simulink model "sim_all"  (R2020a)
settings: Solver=VariableStepAuto  StartTime=0.0  StopTime=2000  RelTol=1e-3
values from neighbouring files (symbols this model uses):
  a1 = rho * D^4 * alpha1    (= 0.000388302366464)    [data_current.m]
  a2 = -rho * D^3 * alpha2 * (1 - omega)    (= 0.0037030698432)    [data_current.m]
  alpha1 = 0.0113    [data_current.m]
  alpha2 = -0.0091    [data_current.m]
  cornerA = [43.781381 ... (first row only)    [missionC.m]
  cornerB = [43.780975 ... (first row only)    [missionC.m]
  cornerC = [43.780189 ... (first row only)    [missionC.m]
  cornerD = [43.780602 ... (first row only)    [missionC.m]
  ctrl_clockwise = false    [controller.m]
  ctrl_int_bound_or = 0.1    [controller.m]
  ctrl_int_bound_pos = 1    [controller.m]
  ctrl_k_or = 1    [controller.m]
  ctrl_k_pos = 1/3    (= 0.333333333333)    [controller.m]
  ctrl_Ki_vel = 100    [controller.m]
  ctrl_Kp_v_pos = 200    [controller.m]
  ctrl_Kp_vel = 200    [controller.m]
  ctrl_TAM = [  1     1           0           0               0       0;               0     0           1           1               0       0;               0     0           0           0               1       1;               0     0  -(ctrl_r+ctrl_dc)  ctrl_r+ctrl_dc    0       0;               0     0           0           0            -ctrl_r    ctrl_r;           -ctrl_r ctrl_r        0           0       ...(+19 chars)    [controller.m]
  ctrl_Ts = 0.1    [controller.m]
  ctrl_va_uncontrolled = 0.15    [controller.m]
  ctrl_vel_uncontrolled = 0.5    [controller.m]
  D = 0.076    [data_current.m]
  dead_zone_limit = 31.5    [data_current.m]
  depth = 5    [missionC.m]
  distanceFromWall = 8    [missionC.m]
  initInspectedSide = 2    [missionC.m]
  initPoint = [ 43.780796 ... (first row only)    [missionC.m]
  mod_A = pi*mod_R*mod_R    [model.m]
  mod_Cd_F = 0.45    [model.m]
  mod_Cd_M = 0.4    [model.m]
  mod_eta_init = [mod_xNorth; mod_yEast; -mod_zDown; 0; 0; 0]    [model.m]
  mod_g = 9.81    [model.m]
  mod_h0 = 0    [model.m]
  mod_Ixx = mod_Io(1,1)    [model.m]
  mod_Iyy = mod_Io(2,2)    [model.m]
  mod_Izz = mod_Io(3,3)    [model.m]
  mod_Kp_dot = 0    [model.m]
  mod_lat0 = 43.780189    [model.m]
  mod_lon0 = 11.282698    [model.m]
  mod_m = 100    [model.m]
  mod_Mq_dot = mod_Kp_dot    (= 0)    [model.m]
  mod_ni_init = [0; 0; 0; 0; 0; 0]    [model.m]
  mod_Nr_dot = mod_Kp_dot    (= 0)    [model.m]
  mod_p1 = [0; mod_R; 0]    [model.m]
  mod_p2 = [0; -mod_R; 0]    [model.m]
  mod_p3 = [0; 0; (mod_R + mod_z_cm)]    [model.m]
  mod_p4 = [0; 0; -(mod_R + mod_z_cm)]    [model.m]
  mod_p5 = [mod_R; 0; 0]    [model.m]
  mod_p6 = [-mod_R; 0; 0]    [model.m]
  mod_R = ((3*mod_Vol)/(4*pi))^(1/3)    [model.m]
  mod_Rm = (4*mod_R)/(3*pi)    [model.m]
  mod_t1 = [1; 0; 0]    [model.m]
  mod_t2 = [1; 0; 0]    [model.m]
  mod_t3 = [0; 1; 0]    [model.m]
  mod_t4 = [0; 1; 0]    [model.m]
  mod_t5 = [0; 0; 1]    [model.m]
  mod_t6 = [0; 0; 1]    [model.m]
  mod_W = mod_m*mod_g    (= 981)    [model.m]
  mod_Xu_dot = (2/3)*mod_rho_AUV*pi*(mod_R^3)    [model.m]
  mod_Yv_dot = mod_Xu_dot    [model.m]
  mod_z_cm = mod_r_cm(3)    [model.m]
  mod_Zw_dot = mod_Xu_dot    [model.m]
  n_max = 340    [data_current.m]
  nav_DT = 0.1    [navigation.m]
  nav_filter = -1    [data_analysis_simulation_total.m]    (also in navigation.m)
  nav_giro = 2    [navigation.m]
  nav_h0 = 0    [navigation.m]
  nav_lat0 = cornerC(1)    [navigation.m]
  nav_lon0 = cornerC(2)    [navigation.m]
  nav_plane_AB = coefficient_plane(nav_A,nav_B)    [navigation.m]
  nav_plane_BC = coefficient_plane(nav_B,nav_C)    [navigation.m]
  nav_plane_CD = coefficient_plane(nav_C,nav_D)    [navigation.m]
  nav_plane_DA = coefficient_plane(nav_D,nav_A)    [navigation.m]
  nav_resampling = 10000    [navigation.m]
  omega = 0.1    [data_current.m]
  relativeDirection = 30    [missionC.m]
  res_enable_n_eff = 1    [navigation.m]
  rho = 1030    [data_current.m]
  sens_distCM = 0.267    [sensors.m]
  sens_Sample_time_AHRS = 0.1    [sensors.m]
  sens_Sample_time_depth = 0.1    [sensors.m]
  sens_Sample_time_dvl = 0.2    [sensors.m]
  sens_Sample_time_GPS = 1    [sensors.m]
  sens_Sample_time_GYRO = 0.1    [sensors.m]
  sens_Sample_time_sonar = 0.5    [sensors.m]
  sens_threshold = 0.485    [sensors.m]
  sens_Variance_AHRS_pitch = (0.0087)^2    (= 7.569e-05)    [sensors.m]
  sens_Variance_AHRS_roll = (0.0087)^2    (= 7.569e-05)    [sensors.m]
  sens_Variance_AHRS_yaw = (0.0017)^2    (= 2.89e-06)    [sensors.m]
  sens_Variance_depth1 = (0.2)^2    (= 0.04)    [sensors.m]
  sens_Variance_depth2 = (0.4)^2    (= 0.16)    [sensors.m]
  sens_Variance_DVL = (speed*0.03)^2    [sensors.m]
  sens_Variance_GPS = 3    [sensors.m]
  sens_Variance_GYRO = 2.5133e-06    [sensors.m]
  sens_Variance_sonar = 0.05    [sensors.m]
  soglia_or = [0.1, 0.1, 0.1]    [mission.m]
  soglia_orp = 0.1    [mission.m]
  soglia_parete = 0.5    [mission.m]
  soglia_parete_frenata = 0.5    [mission.m]
  soglia_pos = [0.00001, 0.00001, 0.5]    [mission.m]
  soglia_SOS_collisione = 2    [mission.m]
  soglia_SOS_or = [0.25, 0.25, 0.25]    [mission.m]
  soglia_SOS_orp = 0.25    [mission.m]
  soglia_SOS_parete = 1    [mission.m]
  soglia_SOS_pos = [0.00005, 0.00005, 1]    [mission.m]
  soglia_SOS_pos_ris = 2    [mission.m]
  soglia_SOS_vel = 0.2    [mission.m]
  SOS = 0    [mission.m]
  speed = 0.4    [missionC.m]
  stato = 100    [mission.m]
  timer = 40*2    (= 80)    [mission.m]
  Ts_supervisor = 0.1    [mission.m]
undefined symbols (not defined in the file or in its folder): DiscIntNeverNeededParam, nav_A, nav_B, nav_C, nav_D
libraries: simulink x8, cstblocks x6, simulink_extras x1
(part 7 of 8)

== matlab function sim_all/Controller_mk4_v3/C_or/C_or_Z ==
  data: err_int output; ang input; vel output; k input; ctrl_va_uncontrolled parameter; ctrl_int_bound_or parameter
%% Azione proporzionale
function [err_int, vel] = fcn(ang, k, ctrl_va_uncontrolled, ctrl_int_bound_or)
    v = 0;
    err_int = 0;
    va_des = ctrl_va_uncontrolled;  % velocità impostata prima della fase di frenata
    brake_dist = (1/k)*va_des;      % distanza in cui dobbiamo iniziare a frenare
    if ang >= brake_dist            % al di fuori dello spazio di frenata
        v = va_des;
    end
    if ang <= -brake_dist           % al di fuori dello spazio di frenata in negativo
        v = -va_des;
    end
    if  abs(ang) < brake_dist       % proporzionale se entro la distanza di frenata
        v = k*ang;
    end
    vel = v;
    if abs(ang) < ctrl_int_bound_or    % per il regime può essere utile una azione integrale
        err_int = ang;                 % err_int va ad un integratore
    end
end

== matlab function sim_all/Controller_mk4_v3/C_pos/C_pos_X ==
  data: err_int output; pos input; vel output; k input; ctrl_vel_uncontrolled parameter; ctrl_int_bound_pos parameter
%% Azione proporzionale
function [err_int, vel] = fcn(pos, k, ctrl_vel_uncontrolled, ctrl_int_bound_pos)
    v = 0;
    err_int = 0;
    vel_des = ctrl_vel_uncontrolled;    % velocità impostata se 'lontani'
    brake_dist = 1/k*vel_des;           % distanza di frenata
    if pos >= brake_dist                % se ho spazio per frenare mantengo la velocità
        v = vel_des;
    end
    if pos <= -brake_dist               % lontani in direzione negativa
        v = -vel_des;
    end
    if  abs(pos) < brake_dist           % se è vicino il proporzionale gestisce la frenata
        v = k*pos;
    end
    vel = v;
    if abs(pos) < ctrl_int_bound_pos    % per il regime può essere utile una azione integrale
        err_int = pos;                  % err_int va ad un integratore
    end

== matlab function sim_all/Controller_mk4_v3/C_pos/C_pos_Z ==
  data: err_int output; pos input; vel output; k input; ctrl_vel_uncontrolled parameter; ctrl_int_bound_pos parameter
%% Azione proporzionale
function [err_int, vel] = fcn(pos, k, ctrl_vel_uncontrolled, ctrl_int_bound_pos)
    v = 0;
    err_int = 0;
    vel_des = ctrl_vel_uncontrolled;    % velocità impostata se 'lontani'
    brake_dist = 1/k*vel_des;           % distanza di frenata
    if pos >= brake_dist                % se ho spazio per frenare mantengo la velocità
        v = vel_des;
    end
    if pos <= -brake_dist               % lontani in direzione negativa
        v = -vel_des;
    end
    if  abs(pos) < brake_dist           % se è vicino il proporzionale gestisce la frenata
        v = k*pos;
    end
    vel = v;
    if abs(pos) < ctrl_int_bound_pos    % per il regime può essere utile una azione integrale
        err_int = pos;                  % err_int va ad un integratore
    end

== matlab function sim_all/PF/Particle Filter/AHRS__check/MATLAB Function4 ==
  data: flag_AHRS output; AHRS_new input; AHRS_now output; AHRS_old input
function [flag_AHRS, AHRS_now] = fcn(AHRS_new, AHRS_old)

    if isnan(AHRS_new(1,1)) || isnan(AHRS_new(2,1)) || isnan(AHRS_new(3,1))
        AHRS_now = AHRS_old;
        flag_AHRS = 1;
        disp('Misura AHRS non valida')
    else
        AHRS_now = AHRS_new;
        flag_AHRS = 0;
    end  
end

== matlab function sim_all/PF/Particle Filter/CORREZIONE/MATLAB Function ==
  data: x_k_1 input; x output; P_k_1 input; s input size=3 1000; w input size=1 1000; flag input; P output; s output; w output; nav_flag_init input
function [x, P, s, w] = correction(x_k_1, P_k_1, s, w, flag,nav_flag_init)

%% -------------------------------------------
    n=1000; 
%% -------------------------------------------

%in base al flag so se i pesi sono stati aggionati o meno nella correzione
%e quindi decido se ricalcolare le x stimate e la P oppure no
       
    x=zeros(3,1); 
    P=zeros(3,3);

    if nav_flag_init ~= 0       %se il filtro è inizializzato
        if flag == 1            %se la correzione è avvenuta ricalcolo x e P
            for i=1:3
                x(i) = sum(w(1,:)*s(i,:)');
            end
            for i=1:n   
              P = P + w(:,i)*((s(:,i)-x)*(s(:,i)-x)');  
            end
        else                    % se la correzione è avvenuta
            x=x_k_1;
            P=P_k_1;
        end
    end
end

== matlab function sim_all/PF/Particle Filter/Creazione vettore delle misure ==
  data: flag_vect output; GPS input; mis_vect output; depth input; s_pr input; s_dx input; s_sx input; mis_vect_prec input; J input; pos input; nav_plane_AB parameter; nav_plane_BC parameter; nav_plane_CD parameter; nav_plane_DA parameter; nav_A parameter; nav_B parameter; nav_C parameter; nav_D parameter; distanceFromWall parameter
%%
% Questa funzione impila le informazioni derivanti dai vari sensori in un
% unico vettore mis_vect 7x1.                                 
% Ci sarà un corrispondente vettore flag_vect 7x1 di flag che sarà pari a:

% flag(i) = 0  se la misura è uguale a quella arrivata nell'istante
% predecente, in tal caso la correzione non verrà effettuata
% flag(i) = 1 se la misura è stata aggiornata rispetto a quella precendente
 
% NB il controllo sulla validità dei dati del GPS è valutata nel blocco
% sucessivo

function [flag_vect,mis_vect] = misure_vector(GPS,depth,s_pr,s_dx,s_sx, mis_vect_prec,...
          J,pos, nav_plane_AB, nav_plane_BC, nav_plane_CD, nav_plane_DA, nav_A, nav_B, nav_C, nav_D, distanceFromWall)
    
    mis_vect = zeros(7,1);
    flag_vect = zeros(7,1);
	mis_vect = [GPS(1) GPS(2) GPS(3) depth s_pr s_dx s_sx]';
    
    for i=[1:7]
        if mis_vect(i) ~= mis_vect_prec(i)
            flag_vect(i) = 1;
        end
    end
    
    %valutiamo se la misura del profondimetro è valida
    if isnan(depth)  
        flag_vect(4) = 0;
    end
     
    %se i dati dei sonar qui sono utilizzabili, dobbiamo assicurarci che il 
    %loro raggio non punti verso uno spigolo, in quel caso potrebbe
    %causare una correzione errata
    
    if flag_vect(5) == 1               %se i dati del sonar di prua sono nuovi
            versore_son_NED = J*[1 0 0]';          %versore terna NED sonar prua
            flag_vect(5) = inter(pos, versore_son_NED ,nav_plane_AB,nav_plane_BC,nav_plane_CD,nav_plane_DA, nav_A, nav_B, nav_C, nav_D);       
    end

    if flag_vect(6) == 1               %se i dati del sonar destro sono nuovi
            versore_son_NED = J*[0 1 0]';          %versore terna NED sonar dx

            flag_vect(6) = inter(pos, versore_son_NED ,nav_plane_AB,nav_plane_BC,nav_plane_CD,nav_plane_DA, nav_A, nav_B, nav_C, nav_D);       
    end
    if flag_vect(7) == 1               %se i dati del sonar sinistro sono nuovi
            versore_son_NED = J*[0 -1 0]';          %versore terna NED sonar sx
            flag_vect(7) = inter(pos, versore_son_NED ,nav_plane_AB,nav_plane_BC,nav_plane_CD,nav_plane_DA, nav_A, nav_B, nav_C, nav_D);
    end 
    %la terza componente di flag_vect non sarà utilizzata. per assicurarci
    %che i dati del GPS siano validi ci rifaremo sempre su mis_vect
    
    
    
    %se il valore del sonar è NaN, non dobbiamo considerare valide le
    %misure, e se il robot troppo lontane dalle pareti
    soglia_distanza=distanceFromWall*3;
    soglia_variazione=0.8;
    if isnan(s_pr) || mis_vect(5) > soglia_distanza || abs(mis_vect(5)- mis_vect_prec(5)) > soglia_variazione
        flag_vect(5) = 0;
    end
    if isnan(s_dx) || mis_vect(6) > soglia_distanza || abs(mis_vect(6)- mis_vect_prec(6)) > soglia_variazione
        flag_vect(6) = 0;
    end
    if isnan(s_sx) || mis_vect(7) > soglia_distanza || abs(mis_vect(7)- mis_vect_prec(7)) > soglia_variazione
        flag_vect(7) = 0;
    end
end




function [flag] = inter(pos, versore_son_NED,nav_plane_AB,nav_plane_BC,nav_plane_CD,nav_plane_DA, nav_A, nav_B, nav_C, nav_D)
    
    %calcolo della distanza dalla posizione ai piani delle pareti seguendo
    %la direzione data dal versore del sonar

    t_AB = -(pos(1)+nav_plane_AB(2)*pos(2)+nav_plane_AB(4))/(nav_plane_AB(2)*versore_son_NED(2)+versore_son_NED(1));
    t_BC = -(pos(1)+nav_plane_BC(2)*pos(2)+nav_plane_BC(4))/(nav_plane_BC(2)*versore_son_NED(2)+versore_son_NED(1));
    t_CD = -(pos(1)+nav_plane_CD(2)*pos(2)+nav_plane_CD(4))/(nav_plane_CD(2)*versore_son_NED(2)+versore_son_NED(1));
    t_DA = -(pos(1)+nav_plane_DA(2)*pos(2)+nav_plane_DA(4))/(nav_plane_DA(2)*versore_son_NED(2)+versore_son_NED(1));
    
    if t_AB < 0
        t_AB = inf;
    end
    if t_BC < 0
        t_BC = inf;
    end
    if t_CD < 0
        t_CD = inf;
    end
    if t_DA < 0
        t_DA = inf;
    end
           
    [dist, index] = min([t_AB t_BC t_CD t_DA]);
    dist = dist - 0.267;       %va tolto il raggio del robot rispetto al centro di massa
    
    int=zeros(1,3);
    %calcolo l'intersezione
    int(1) = pos(1) + versore_son_NED(1)*dist;
    int(2) = pos(2) + versore_son_NED(2)*dist;
    int(3) = 0;
    
    
    
    soglia_spigolo = 5;          %distanza massima dallo spigolo entro la quale 
                       %la misura del sonar non è buona
    flag=1;
    switch index
        case 1      
            if norm(int-nav_A) < soglia_spigolo || norm(int-nav_B) < soglia_spigolo
                flag=0;
            end
        case 2
            if norm(int-nav_B) < soglia_spigolo || norm(int-nav_C) < soglia_spigolo
                flag=0;
            end
        case 3
            if norm(int-nav_C) < soglia_spigolo || norm(int-nav_D) < soglia_spigolo
                flag=0;
            end
        case 4
            if norm(int-nav_D) < soglia_spigolo || norm(int-nav_A) < soglia_spigolo
                flag=0;
            end
        otherwise
            disp('errore nella intersezione del piano')
    end
end

== matlab function sim_all/Mission_supervisor_v3/Mission_Supervisor/MATLAB Function1 ==
  data: punto_iniz_patt output size=3; initInspectedSide parameter; distanceFromWall parameter; initPoint parameter; Or_in output; dps_fin output; cornerA parameter; cornerB parameter; cornerC parameter; cornerD parameter; relativeDirection parameter; alfa output
function [punto_iniz_patt, Or_in, dps_fin, alfa] = ambiente(initInspectedSide,distanceFromWall,initPoint,cornerA, cornerB, cornerC, cornerD, relativeDirection)
 
    %% Unità di misura 
    
    % punto_iniz_patt, initPoint, cornerA, cornerB, cornerC, cornerD        [deg, deg, m]
    % Or_in                                                                 [rad, rad, rad]
    % dps_fin,distanceFromWall                                              [m]
    % alfa                                                                  [rad]
    % relativeDirection                                                     [deg]

    %% Inizializzazione variabili
    
    % Valori dati da file relativi agli angoli del bacino
    iP = initPoint;
    A = cornerA;
    B = cornerB;
    C = cornerC;
    D = cornerD;

    coder.extrinsic('evalin', 'wgs84Ellipsoid', 'geodetic2ned');
    coder.extrinsic('evalin', 'wgs84Ellipsoid', 'ned2geodetic');

    % Inizializzazione di alcune variabili
    xA = 0; yA = 0; zA = 0; xB = 0; yB = 0; zB = 0; xC = 0; yC = 0; zC = 0; 
    xD = 0; yD = 0; zD = 0; xiP = 0; yiP = 0; ziP = 0;
    xpipAB = 0; ypipAB = 0; zpipAB = 0; xpipBC = 0; ypipBC = 0; zpipBC = 0; 
    xpipCD = 0; ypipCD = 0; zpipCD = 0; xpipDA = 0; ypipDA = 0; zpipDA = 0;
    depth_in = initPoint(3);
    Or_in = [0; 0; 0];
    
    % Conversione da Geodetic a NED delle posizioni degli angoli e del punto iniziale
    wgs84 = wgs84Ellipsoid; % Per il corretto funzionamento e' necessario installare un 
                            % pacchetto aggiuntivo in Matlab qualora non fosse presente
    [xA, yA, zA] = geodetic2ned(A(1), A(2), 0, C(1), C(2), 0, wgs84);
    [xB, yB, zB] = geodetic2ned(B(1), B(2), 0, C(1), C(2), 0, wgs84);
    [xC, yC, zC] = geodetic2ned(C(1), C(2), 0, C(1), C(2), 0, wgs84);
    [xD, yD, zD] = geodetic2ned(D(1), D(2), 0, C(1), C(2), 0, wgs84);
    [xiP, yiP, ziP] = geodetic2ned(iP(1), iP(2), 0, C(1), C(2), 0, wgs84);
    inizio = [xiP; yiP; depth_in];

    % Punti centrali delle pareti
    pcAB = [(xB + xA)/2; (yB + yA)/2; depth_in];
    pcBC = [(xB + xC)/2; (yB + yC)/2; depth_in];   
    pcCD = [(xC + xD)/2;(yC + yD)/2; depth_in];
    pcDA = [(xD + xA)/2; (yD + yA)/2; depth_in];

    % Lunghezze delle pareti
    AB = sqrt((xA - xB)^2 + (yA - yB)^2); 
    BC = sqrt((xB - xC)^2 + (yB - yC)^2); 
    CD = sqrt((xC - xD)^2 + (yC - yD)^2); 
    DA = sqrt((xD - xA)^2 + (yD - yA)^2); 
    
    dW = distanceFromWall;

    %% Calcolo punto di inizio pattugliamento a meta' parete

    % Calcolo degli angoli relativi tra le pareti 
    thetaBC = acos(yB/BC);          
    thetaCD = acos(yD/CD);
    gammaAB = acos((yB - yA)/AB);
    thetaAB = pi - gammaAB;
    gammaDA = acos((yA - yD)/DA);

    % Punti di inizio pattugliamento a seconda di quale parete è scelta come
    % parete iniziale
    
    dbpc = sqrt((pcAB(1) - xB)^2 + (pcAB(2) - yB)^2);
    hpb = sqrt(dbpc^2 + dW^2);
    alfa1 = - acos(dbpc/hpb);
    gammaab = pi - (gammaAB + alfa1);
    pcab1 = [hpb * sin(gammaab), hpb * cos(gammaab)];
    pipAB = [xB + pcab1(1); yB + pcab1(2); depth_in];

    dcpc = sqrt(pcBC(1)^2 + pcBC(2)^2);
    hpc = sqrt(dcpc^2 + dW^2);
    alfabc = acos(dcpc/hpc);
    gammaBC = thetaBC + alfabc;
    pipBC = [hpc * sin(gammaBC); hpc * cos(gammaBC); depth_in];

    dcdpc = sqrt(pcCD(1)^2 + pcCD(2)^2);
    hpcd = sqrt(dcdpc^2 + dW^2);
    alfacd = acos(dcdpc/hpcd);
    gammaCD = thetaCD - alfacd;
    pipCD = [hpcd * sin(gammaCD); hpcd * cos(gammaCD); depth_in];

    dapc = sqrt((pcDA(1) - xA)^2 + (pcDA(2) - yA)^2);
    hpda = sqrt(dapc^2 + dW^2);
    alfada = acos(dapc/hpda);
    gammada = pi + (gammaDA + alfada);
    pcda1 = [hpda * sin(gammada), hpda * cos(gammada)];
    pipDA = [xA + pcda1(1); yA + pcda1(2); depth_in];
    
    % Si convertono i punti "pip" da NED a Geodetic 
    [xpipAB, ypipAB, zpipAB] = ned2geodetic(pipAB(1), pipAB(2), pipAB(3), C(1), C(2), 0, wgs84);
    [xpipBC, ypipBC, zpipBC] = ned2geodetic(pipBC(1), pipBC(2), pipBC(3), C(1), C(2), 0, wgs84);
    [xpipCD, ypipCD, zpipCD] = ned2geodetic(pipCD(1), pipCD(2), pipCD(3), C(1), C(2), 0, wgs84);
    [xpipDA, ypipDA, zpipDA] = ned2geodetic(pipDA(1), pipDA(2), pipDA(3), C(1), C(2), 0, wgs84);

    pipAB_geodetic = [xpipAB; ypipAB; depth_in];
    pipBC_geodetic = [xpipBC; ypipBC; depth_in];
    pipCD_geodetic = [xpipCD; ypipCD; depth_in];
    pipDA_geodetic = [xpipDA; ypipDA; depth_in];

    %% Calcolo angolo di orientazione iniziale in direzione del punto di inizio  pattugliamento (rispetto al nord)

    % Versore orinetato verso il nord n = [1, 0, 0];
    
    % Vettori che vanno dal punto di partenza al punto di inizio pattugliamento
    
    iAB = pipAB - inizio;
    iBC = pipBC - inizio;
    iCD = pipCD - inizio;
    iDA = pipDA - inizio;

    % Angoli tra direzione Nord e il vettore che porta verso il punto di inizio pattugliamento. 
    % Sono gli angoli di orientazione iniziale desiderata. 
    theta1 = atan2d(iAB(2),iAB(1));
    theta2 = atan2d(iBC(2),iBC(1));
    theta3 = atan2d(iCD(2),iCD(1));
    theta4 = atan2d(iDA(2),iDA(1));
    
    % Si raccoglie in un vettore
    theta = [deg2rad(theta1), deg2rad(theta2), deg2rad(theta3), deg2rad(theta4)];

    %% Si calcolano gli angoli interni dei vertici
    
    alfaC = thetaCD - thetaBC;
    alfaB = pi - (thetaAB-thetaBC);
    alfaA = thetaAB - gammaDA;
    alfaD = 2*pi - alfaA - alfaB - alfaC;
    alfa = [alfaA; alfaB; alfaC; alfaD];    %Utilizzati poi in fase di manovra

    %% Calcolo distanza dalla parete successiva a partire da meta'  parete

    % Sono le distanze da metà parete alla parete successiva
    dABpc = sqrt((pcAB(1) - xB)^2 + (pcAB(2) - yB)^2);
    dBCpc = sqrt(pcBC(1)^2 + pcBC(2)^2);
    dCDpc = sqrt(pcCD(1)^2 + pcCD(2)^2);
    dDApc = sqrt((pcDA(1) - xA)^2 + (pcDA(2) - yA)^2);


    %% Scelta delle condizioni

    % In base al valore di parete iniziale si assegnano i giusti valori per i 
    % riferimenti da utilizzare nei vari stati
    
    if initInspectedSide == 1

        punto_iniz_patt = pipAB_geodetic;
        Or_in = [0; 0; theta(1)];
        dps_fin = dABpc;

    elseif initInspectedSide == 2

        punto_iniz_patt = pipBC_geodetic;
        Or_in = [0; 0; theta(2)];
        dps_fin = dBCpc;

    elseif initInspectedSide == 3

        punto_iniz_patt = pipCD_geodetic;
        Or_in = [0; 0; theta(3)];
        dps_fin = dCDpc;

    else

        punto_iniz_patt = pipDA_geodetic;
        Or_in = [0; 0; theta(4)];
        dps_fin = dDApc;

    end
                                                                            %****TEST*****%
                                                                            %Or_in = [1; 1; 1];

end

== matlab function sim_all/PF/Particle Filter/DVL_check/MATLAB Function4 ==
  data: flag_DVL output; DVL_new input; DVL_now output; DVL_old input
function [flag_DVL, DVL_now] = fcn(DVL_new, DVL_old)

    if isnan(DVL_new(1,1)) || isnan(DVL_new(2,1)) || isnan(DVL_new(3,1))
        DVL_now = DVL_old;
        flag_DVL = 1;
        disp('Misura DVL non valida')
    else
        DVL_now = DVL_new;
        flag_DVL = 0;
    end  
end

== matlab function sim_all/Controller_mk4_v3/InputOr_Organizer/diff_or ==
  data: or_d input; err_or output; or_s input
%% Calcolo errore
function err_or = fcn(or_d, or_s)
coder.extrinsic('wrapToPi');
err_or = zeros(3,1);
err_or = wrapToPi(or_d - or_s);    % rimane compreso tra -pi e +pi
end

== matlab function sim_all/Controller_mk4_v3/InputPos_Organizer/Ned2Body1 ==
  data: x_n input size=[3 1]; x_b output size=[3 1]; or input
%% Da NED a BODY
function x_b = ned2body(x_n,or)
C=zeros(3,3);
C=Cx(or(1))'*Cy(or(2))'*Cz(or(3))';
x_b = C'*x_n;
end

== matlab function sim_all/PF/Particle Filter/Inizializzazione Filtro ==
  data: GPS input; s0 output size=3 1000; depth input; w0 output size=1 1000; flag input; flag output; sens_Variance_GPS parameter; sens_Variance_depth1 parameter


function [s0, w0, flag] = PF_init(GPS, depth, flag, sens_Variance_GPS, sens_Variance_depth1)
%% -------------------------------------------
    n=1000; 
%% -------------------------------------------
    s0 = zeros(3,n);
    w0 = 1/n*ones(1,n);
    
    % il valore di nav_flag_init è all'inizio della simulazione pari a 0
    % appena c'è il primo dato disponibile del GPS (insieme al profondimetro)
    % si assume quella come punto di inizializzazione delle particelle.

    if flag == 0
        if GPS(3)==1
        GPS_w_x = sqrt(sens_Variance_GPS).*randn(n,1);
        GPS_w_y = sqrt(sens_Variance_GPS).*randn(n,1);
        depth_w = sqrt(sens_Variance_depth1).*randn(n,1);
            for i=1:n
                s0(:,i) = s0(:,i) + [GPS(1)+GPS_w_x(i), GPS(2)+GPS_w_y(i), depth+depth_w(i)]';
            end
            flag = 1;            %se vale 1 bisogna assegnare i primi valori a s
        end
               
    end

end

== matlab function sim_all/PF/Particle Filter/MATLAB Function1 ==
  data: orient input; J output
function J = calcolo_J(orient)

    Roll  = orient(1);
    Pitch = orient(2);
    Yaw   = orient(3);

    R_x = [ 1               0              0;
            0           cos(Roll)     sin(Roll);
            0           -sin(Roll)    cos(Roll)];

    R_y = [cos(Pitch)       0   -sin(Pitch);
              0             1         0;
           sin(Pitch)       0   cos(Pitch)];

    R_z = [cos(Yaw)     sin(Yaw)      0;
          -sin(Yaw)     cos(Yaw)      0;
              0            0          1];

    J = (R_z'*R_y')*R_x';
end

== matlab function sim_all/PF/Particle Filter/MATLAB Function5 ==
  data: u input; dev_standard_x output; dev_standard_y output; dev_standard_z output
function [dev_standard_x,dev_standard_y,dev_standard_z] = fcn(u) 
    
    dev_standard_x = sqrt(u(1,1));
    dev_standard_y = sqrt(u(2,2));
    dev_standard_z = sqrt(u(3,3));
end

== matlab function sim_all/Controller_mk4_v3/InputPos_Organizer/Ned2Body2 ==
  data: x_n input size=[3 1]; x_b output size=[3 1]; or input
%% Da NED a BODY
function x_b = ned2body(x_n,or)
C=zeros(3,3);
C=Cx(or(1))'*Cy(or(2))'*Cz(or(3))';
x_b = C'*x_n;
end

== matlab function sim_all/EKF/Extended Kalman Filter/MATLAB Function5 ==
  data: u input; dev_standard_x output; dev_standard_y output; dev_standard_z output
function [dev_standard_x,dev_standard_y,dev_standard_z] = fcn(u) 
    
    dev_standard_x = sqrt(u(1,1));
    dev_standard_y = sqrt(u(2,2));
    dev_standard_z = sqrt(u(3,3));
end

== matlab function sim_all/Controller_mk4_v3/InputPos_Organizer/Ned2Body3 ==
  data: x_n input size=[3 1]; x_b output size=[3 1]; or input
%% Da NED a BODY
function x_b = ned2body(x_n,or)
C=zeros(3,3);
C=Cx(or(1))'*Cy(or(2))'*Cz(or(3))';
x_b = C'*x_n;
end

== matlab function sim_all/Controller_mk4_v3/InputPos_Organizer/Ned2Body4 ==
  data: x_n input size=[3 1]; x_b output size=[3 1]; or input
%% Da NED a BODY
function x_b = ned2body(x_n,or)
C=zeros(3,3);
C=Cx(or(1))'*Cy(or(2))'*Cz(or(3))';
x_b = C'*x_n;
end

== matlab function sim_all/Controller_mk4_v3/InputPos_Organizer/brake_trigger ==
  data: state input; trigg_brake output
%% Restituisce 0 se in frenata
% In frenata vengono controllate sia dpp che dps
function trigg_brake = fcn(state)
tmp = 0;
switch state
    case 100            % fermo in superficie
        tmp = 1;
    case 101            % orientazione verso parete di inizio in superficie
        tmp = 1;
    case 102            % posizionamento in superficie
        tmp = 1;   
    case 103            % immersione
        tmp = 1;
    case 104            % orientazione in profondità
        tmp = 1;
    case 201            % pattugliamento
        tmp = 1;
    case 202            % frenata
        tmp = 0;
    case 203            % manovra di cambio parete
        tmp = 0;
    case 204            % competamento del pattugliamento della parete iniziale
        tmp = 1;
    case 205            % frenata a metà parete
        tmp = 0;
    case 301            % risalita
        tmp = 0;
    case 302            % orientazione in superficie
        tmp = 1;
    case 303            % rientro, ritorno al punto iniziale in superficie
        tmp = 1;
    case 304            % fine missione, tutto spento
        tmp = 1;
end
trigg_brake = tmp;
end

== matlab function sim_all/Controller_mk4_v3/InputVel_Organizer/Ned2Body4 ==
  data: x_n input size=[3 1]; x_b output size=[3 1]; or input
%% Da NED a BODY
function x_b = ned2body(x_n,or)
C=zeros(3,3);
C=Cx(or(1))'*Cy(or(2))'*Cz(or(3))';
x_b = C'*x_n;
end

== matlab function sim_all/Controller_mk4_v3/Mixer/Mix ==
  data: Tp input; T output; Tv input; To input; ctrl_T_max parameter
%% funzione che permette di gestire le saturazioni dei motori
function T = Mix(Tp, Tv, To, ctrl_T_max)
    T_sat = [   ctrl_T_max   ctrl_T_max   ctrl_T_max   ctrl_T_max   ctrl_T_max   ctrl_T_max;...
               -ctrl_T_max  -ctrl_T_max  -ctrl_T_max  -ctrl_T_max  -ctrl_T_max  -ctrl_T_max];
    tmp = Tp + Tv + To;
    freg = sumSat(ctrl_T_max, tmp);                 % freg indica se il vettore è da regolare
    if freg == true
        if sumSat(ctrl_T_max, To+Tp) == false       % caso in cui To+Tp non satura
            T_tmp = To + Tp;
            [T_sat, T_new] = prior(T_sat, T_tmp);
            [T_sat, T_new] = prior(T_sat, Tv);
            T = T_tmp + T_new;
        else                                        % caso generale, ridimensiona tutti i vettori che fanno saturare
            T_tmp = 0;
            [T_sat, T_new] = prior(T_sat, To);
            T_tmp = T_tmp + T_new;
            [T_sat, T_new] = prior(T_sat, Tp);
            T_tmp = T_tmp + T_new;
            [T_sat, T_new] = prior(T_sat, Tv);
            T = T_tmp + T_new;
        end
    else
        T = tmp;
    end
end

% sumSat() restituisce 1 se il vettore T_in supera la saturazione, è solo
% un controllo iniziale in quanto controlla solo se la somma delle spinte
% rientra in T_max
function resp = sumSat(T_max, T_in)
    tmp = false;
    for i=1:length(T_in)
        if abs(T_in(i)) > T_max
            tmp = true;
        end
    end
    resp = tmp;
end

% prior() prende vettore in ingresso e vettore delle saturazioni e
% restituisce vettore in ingresso ridimensionato e nuovo vettore delle
% saturazioni
function [T_sat_new, T_reg] = prior(T_sat, T_new)
    T_sat_tmp = T_sat;
    recalc = false;                 % serve per sapere se bisogna ricalcolare le precedenti saturazioni
    for i = 1:length(T_new)         % ciclo per calcolare i nuovi vettori ridimensionati
        if T_new(i)>0               % azione del motore positiva
            tmp = T_sat_tmp(1,i) - T_new(i);        % nuova saturazione temporanea
            if tmp < 0
                if i < 5                            % devo scalare i primi 4 motori per mantenere la direzione
                    k = abs(T_sat_tmp(1,i)/T_new(i));
                    T_new(1:4) = T_new(1:4) * k;
                    if i~=1                 % devo riaggiustare le T_sat precedenti se il motore che satura non è il primo
                        recalc = true;      % riaggiusto i T_sat in prior2
                    end
                else
                    k = abs(T_sat_tmp(1,i)/T_new(i));
                    j = ((floor(i/2.1)+1)*2);           % escamotage per prendere le coppie giuste, era per le coppie
                    T_new(j-1:j) = T_new(j-1:j) * k;    % ridimensiono le componenti relative al grado di libertà
                    if mod(i, 2) == 0                   % devo riaggiustare la T_sat precedente se i pari
                        recalc = true;                  % riaggiusto gli T_sat
                    end
                end
            end
            T_sat_tmp(1,i) = T_sat_tmp(1,i) - T_new(i);
            T_sat_tmp(2,i) = T_sat_tmp(2,i) - T_new(i);
        elseif T_new(i)<0                           % è identico al codice per T>0 ma speculare
            tmp = T_sat_tmp(2,i) - T_new(i);
            if tmp > 0
                if i < 5                            % devo scalare i primi 4 motori
                    k = abs(T_sat_tmp(2,i)/T_new(i));
                    T_new(1:4) = T_new(1:4) * k;
                    if i~=1                         % devo riaggiustare le T_sat precedenti se i 
                        recalc = true;              % riaggiusto gli T_sat
                    end
                else
                    k = abs(T_sat_tmp(2,i)/T_new(i));
                    j = (floor(i/2.1)+1)*2;     % escamotage per prendere le coppie giuste
                    T_new(j-1:j) = T_new(j-1:j) * k;
                    if mod(i, 2) == 0           % devo riaggiustare la T_sat precedente se i pari
                        recalc = true;          % riaggiusto gli T_sat
                    end
                end
            end
            T_sat_tmp(2,i) = T_sat_tmp(2,i) - T_new(i);
            T_sat_tmp(1,i) = T_sat_tmp(1,i) - T_new(i);
        end
    end
    if recalc == true
        % devo rifare il ciclo con i nuovi T_new
        [T_sat_tmp, T_new] = prior2(T_sat, T_new);
    end
    T_sat_new = T_sat_tmp;      % T_sat_new è il nuovo vettore delle saturazioni
    T_reg = T_new;              % T_reg è il nuovo vettore scalato
end

% prior2() aggiusta il vettore delle saturazioni T_sat, uso interno a
% prior()
function [T_sat_new, T_reg] = prior2(T_sat, T_new)
    T_sat_tmp = T_sat;
    for i = 1:length(T_new)        % ciclo per calcolare quanti giri rimanenti prima di saturare
        if T_new(i)>0              % azione del motore positiva
            tmp = T_sat_tmp(1,i) - T_new(i);       % nuova saturazione temporanea
            T_sat_tmp(1,i) = tmp;
            T_sat_tmp(2,i) = T_sat_tmp(2,i) - T_new(i);
        else
            tmp = T_sat_tmp(2,i) - T_new(i);
            T_sat_tmp(2,i) = tmp;
            T_sat_tmp(1,i) = T_sat_tmp(1,i) - T_new(i);
        end
    end
    T_sat_new = T_sat_tmp;
    T_reg = T_new;
end

== matlab function sim_all/Controller_mk4_v3/Mixer/T2n ==
  data: T input size=[6 1]; n output; a1 parameter
%% Conversione da T a n
% Si usa relazione inclusa nel modello dei propulsiori
% sfruttando approssimazione quadratica
function n = T2n(T,a1)
n = zeros(6,1);
    for i= 1:length(T)
        if T(i) > 0
            n(i) = sqrt(T(i)/a1);
        else
            n(i) = -sqrt(-T(i)/a1);
        end
    end
end

== matlab function sim_all/Controller_mk4_v3/enabler ==
  settings: updateMethod=DISCRETE  sampleTime=ctrl_Ts
  data: state input; en_pos output; en_vel output; en_or output
function [en_pos, en_vel, en_or] = fcn(state)
    en = [0 0 0];
    persistent state_prec        % reset dell'azione integrale
    if isempty(state_prec)
        state_prec = 0;
    end
    if state ~= state_prec
        en = [0 0 0];
        state_prec = state;
    else
        switch state
            case 100            % fermo in superficie
                en = [1 0 0];
            case 101            % orientazione verso parete di inizio in superficie
                en = [1 0 1];
            case 102            % posizionamento in superficie
                en = [1 0 1];   
            case 103            % immersione
                en = [1 0 1];
            case 104            % orientazione in profondità
                en = [1 0 1];
            case 201            % pattugliamento
                en = [1 1 1];
            case 202            % frenata, da verificare con gli altri
                en = [1 0 1];
            case 203            % manovra di cambio parete
                en = [1 0 1];
            case 204            % competamento del pattugliamento della parete iniziale
                en = [1 1 1];
            case 205            % frenata a metà parete
                en = [1 0 1];
            case 301            % risalita
                en = [1 0 1];
            case 302            % orientazione in superficie
                en = [1 0 1];
            case 303            % rientro, ritorno al punto iniziale in superficie
                en = [1 0 1];
            case 304            % fine missione, tutto spento
                en = [0 0 0];
        end
    end
    en_pos = en(1);
    en_vel = en(2);
    en_or = en(3);
end

== matlab function sim_all/Controller_mk4_v3/lld2Ned ==
  data: x_ecef input size=[3 1]; x_n output; cornerC parameter
%% Da LLD (riferimento posizione assoluta) a NED
function x_n = ToNed_Pos(x_ecef,cornerC)
x_n=zeros(3,1);
coder.extrinsic('evalin', 'wgs84Ellipsoid', 'geodetic2ned');
[pNorth,pEast,pDown] = geodetic2ned(x_ecef(1),x_ecef(2),x_ecef(3),cornerC(1),cornerC(2),0,wgs84Ellipsoid);
x_n=[pNorth;pEast;x_ecef(3)];

end

== matlab function sim_all/PF/Particle Filter/MISURA VIRTUALE/MATLAB Function ==
  data: s input size=3 1000; w_k output size=1 1000; w input size=1 1000; flag_vect input; mis_vect input; J input; R input; flag output size=1; nav_plane_AB parameter; nav_plane_BC parameter; nav_plane_CD parameter; nav_plane_DA parameter
function [w_k, flag] = virtual_meas(s, w, flag_vect, mis_vect, J, R,nav_plane_AB, nav_plane_BC, nav_plane_CD, nav_plane_DA)

%% -------------------------------------------
    n=1000; 
%% -------------------------------------------

% che misure darebbero i sensori se fossimo nello stato descritto da s?
    e = zeros(6,n);
    h = zeros(6,n);
    z = zeros(6,n);
    n_sens=0;           %tiene traccia del numero di sensori usati per la correzione
    
    

    %valutazione misure GPS
    if mis_vect(3)==1                                   %se i dati del GPS sono validi
        if flag_vect(1) == 1 && flag_vect(2) == 1       %se i dati del GPS sono nuovi
            for i=1:n
                z(:,i) = z(:,i) + [mis_vect(1) mis_vect(2) 0 0 0 0]';
                h(:,i) = h(:,i) + [   s(1,i)     s(2,i)    0 0 0 0]';
                n_sens=n_sens+2;
            end
        end
    end

    %valutazione misure depth
    if flag_vect(4) == 1                                 %se i dati del profondimetro sono nuovi
        for i=1:n
            z(:,i) = z(:,i) + [0 0 mis_vect(4) 0 0 0]'; 
            h(:,i) = h(:,i) + [0 0    s(3,i)   0 0 0]';
            n_sens=n_sens+1;
        end
    end

    %valutiamo ora le misure virtuali solo se quelle del GPS non sono
    %valide
    if mis_vect(3)==0                      %se i dati del GPS non sono validi

        if flag_vect(5) == 1               %se i dati del sonar di prua sono nuovi
            for i=1:n
                versore_son_NED = J*[1 0 0]';          %versore terna NED sonar prua
                distanza = inter(s(:,i), versore_son_NED ,nav_plane_AB,nav_plane_BC,nav_plane_CD,nav_plane_DA);
                z(:,i) = z(:,i) + [0 0 0 mis_vect(5) 0 0]'; 
                h(:,i) = h(:,i) + [0 0 0 distanza    0 0]';
                n_sens=n_sens+1;
            end
        end

        if flag_vect(6) == 1               %se i dati del sonar destro sono nuovi
            for i=1:n
                versore_son_NED = J*[0 1 0]';          %versore terna NED sonar dx
                distanza = inter(s(:,i), versore_son_NED ,nav_plane_AB,nav_plane_BC,nav_plane_CD,nav_plane_DA);
                z(:,i) = z(:,i) + [0 0 0 0 mis_vect(6) 0]'; 
                h(:,i) = h(:,i) + [0 0 0 0 distanza    0]';
                n_sens=n_sens+1;
            end
        end

        if flag_vect(7) == 1               %se i dati del sonar sinistro sono nuovi
            for i=1:n
                versore_son_NED = J*[0 -1 0]';          %versore terna NED sonar sx
                distanza = inter(s(:,i), versore_son_NED ,nav_plane_AB,nav_plane_BC,nav_plane_CD,nav_plane_DA);
                z(:,i) = z(:,i) + [0 0 0 0 0 mis_vect(7)]'; 
                h(:,i) = h(:,i) + [0 0 0 0 0 distanza   ]';
                n_sens=n_sens+1;
            end
        end
    end
    
    e = z - h;
    n_sens = n_sens/n;
    
   %%riduco le dimensioni della matrice R e del vettore e
    R_rid=R;
    i=0;
    if mis_vect(3) == 0                    %se i dati del GPS non sono validi
        R_rid(1-i,:) = [];
        R_rid(:,1-i) = [];
        e(1-i,:) = [];
        i=i+1;
        R_rid(2-i,:) = [];
        R_rid(:,2-i) = [];
        e(2-i,:) = [];
        i=i+1;
        if flag_vect(4) == 0               %se i dati del profondimetro non sono nuovi
            R_rid(3-i,:) = [];
            R_rid(:,3-i) = [];
            e(3-i,:) = [];
            i=i+1;
        end
        if flag_vect(5) == 0               %se i dati del sonar di prua non sono nuovi
            R_rid(4-i,:) = [];
            R_rid(:,4-i) = [];
            e(4-i,:) = [];
            i=i+1;
        end
        if flag_vect(6) == 0               %se i dati del sonar sinistro non sono nuovi
            R_rid(5-i,:) = [];
            R_rid(:,5-i) = [];
            e(5-i,:) = [];
            i=i+1;
        end
        if flag_vect(7) == 0               %se i dati del sonar destro non sono nuovi
            R_rid(6-i,:) = [];
            R_rid(:,6-i) = [];
            e(6-i,:) = [];
        end
    % da qui invece abbiamo il GPS valido
    else
        if flag_vect(1)==0 || flag_vect(2)==0  %se i dati del GPS non sono nuovi
            R_rid(1-i,:) = [];
            R_rid(:,1-i) = [];
            e(1-i,:) = [];
            i=i+1;
            R_rid(2-i,:) = [];
            R_rid(:,2-i) = [];
            e(2-i,:) = [];
            i=i+1;
        end
        
        if flag_vect(4) == 0               %se i dati del profondimetro non sono nuovi
            R_rid(3-i,:) = [];
            R_rid(:,3-i) = [];
            e(3-i,:) = [];
            i=i+1;
        end
        
        R_rid(4-i,:) = [];                      %annulliamo le misure dei sonar
        R_rid(:,4-i) = [];
        e(4-i,:) = [];
        i=i+1;
        R_rid(5-i,:) = [];
        R_rid(:,5-i) = [];
        e(5-i,:) = [];
        i=i+1;
        R_rid(6-i,:) = [];
        R_rid(:,6-i) = [];
        e(6-i,:) = [];
    end
    
    %% Calcolo la likelihood di ogni particella con e, R n_sens
    %uso la formula della probabilità congiunta in caso di variabili
    %vettoriali
    w_ = zeros(1,n);
    if n_sens ~= 0
        likelihood = zeros(1,n);
        for i=1:n
            esp = e(:,i)'*inv(R_rid)*e(:,i);
            likelihood(i) = exp(-0.5*esp) / (sqrt((2*pi)^n_sens * det(R_rid)));      
        end
        w_= w;
        w_ = w_.*likelihood;
        w_k = w_/sum(w_);

        flag = 1;
    else
        w_k = w;
        flag = 0;
    end
end

%%
%%%%%%%%%%%%%%%%%%%%%%%%%%%%%%%%%%%%%%%%%%%%%%%%%%%%%%%%%%%%%%%%%%%%%%%%%%%%%%%%%%%%%%%%

function [dist] = inter(pos, versore_son_NED,nav_plane_AB,nav_plane_BC,nav_plane_CD,nav_plane_DA)
    
    %calcolo della distanza dalla posizione ai piani delle pareti seguendo
    %la direzione data dal versore del sonar

    t_AB = -(pos(1)+nav_plane_AB(2)*pos(2)+nav_plane_AB(4))/(nav_plane_AB(2)*versore_son_NED(2)+versore_son_NED(1));
    t_BC = -(pos(1)+nav_plane_BC(2)*pos(2)+nav_plane_BC(4))/(nav_plane_BC(2)*versore_son_NED(2)+versore_son_NED(1));
    t_CD = -(pos(1)+nav_plane_CD(2)*pos(2)+nav_plane_CD(4))/(nav_plane_CD(2)*versore_son_NED(2)+versore_son_NED(1));
    t_DA = -(pos(1)+nav_plane_DA(2)*pos(2)+nav_plane_DA(4))/(nav_plane_DA(2)*versore_son_NED(2)+versore_son_NED(1));
    
    if t_AB < 0
        t_AB = inf;
    end
    if t_BC < 0
        t_BC = inf;
    end
    if t_CD < 0
        t_CD = inf;
    end
    if t_DA < 0
        t_DA = inf;
    end
           
    dist = min([t_AB t_BC t_CD t_DA]);
    dist = dist - 0.267;       %va tolto il raggio del robot rispetto al centro di massa
end

== matlab function sim_all/PF/Particle Filter/PREDIZIONE/MATLAB Function ==
  data: x output size=3 1; P output size=3 3; s0 input size=3 1000; w0 input size=1 1000; s input size=3 1000; w input size=1 1000; s output; orient input; DVL input; Q input; nav_DT parameter; nav_flag_init input; w output; nav_flag_init output
%% PREDIZIONE
% parametri in ingresso:
% -   s0     = matrice 3xn particelle iniziali
% -   w0     = matrice 3xn pesi iniziali
% -   s      = matrice 3xn particelle istante precedente
% -   w      = matrice 3xn pesi istante precedente
% -   orient = vettore 3x1 (colonna) dall'AHRS
% -   DVL    = vettore 3x1 (colonna) dal DVL


% parametri in uscita:
% -   x      = vettore 3x1 dello stato
% -   P      = vettore 3x3 delle varianze dello stato
% -   s      = matrice 3xn particelle istante precedente
% -   w      = matrice 3xn pesi istante precedente

function [x, P, s, w, nav_flag_init] = prediction(s0, w0, s, w, orient, DVL, Q, nav_DT, nav_flag_init)
    
%% ------------------------------------------
    n=1000; 
%% -------------------------------------------

    x=zeros(3,1); 
    P=zeros(3,3);
    
    if nav_flag_init ~= 0      
        if nav_flag_init == 1
            s = s0;
            w = w0;
            nav_flag_init = 2;      % =2 così l'inizializzazione è fatta una sola volta.
        end
        
        %genero i vettori di DVL e AHRS sporcati dal rumore per la
        %propagazione delle particelle
        Q_orient = diag([Q(1,1) Q(2,2) Q(3,3)]);
        Q_DVL = diag([Q(4,4) Q(5,5) Q(6,6)]);
        orient_w=zeros(3,n);
        DVL_w=zeros(3,n);
        orient_err = sqrt(Q_orient)*randn(3,n);
        DVL_err = sqrt(Q_DVL)*randn(3,n);
        for i=1:n
            orient_w(:,i) = orient + orient_err(:,i);    %dim 3xn
            DVL_w(:,i) = DVL +  DVL_err(:,i) ;          %dim 3xn
        end

        %applico la f ai campioni
        for i = 1:n
            J = calcolo_J(orient_w);                %devo calcolarla n volte!
            s(:,i) = s(:,i) + nav_DT * J * DVL_w(:,i);   
        end
        %calcolo stato e covarianza dalle particelle e dai pesi
        for i=1:3
            x(i) = sum(w(1,:)*s(i,:)');
        end
        for i=1:n   
              P = P + w(:,i)*((s(:,i)-x)*(s(:,i)-x)');  
        end
    end
end




%% Funzione per il calcolo della matrice di rotazione J

function J = calcolo_J(orient)
    Roll  = orient(1);
    Pitch = orient(2);
    Yaw   = orient(3);
    R_x = [ 1               0              0;
            0           cos(Roll)     sin(Roll);
            0           -sin(Roll)    cos(Roll)];
    R_y = [cos(Pitch)       0   -sin(Pitch);
              0             1         0;
           sin(Pitch)       0   cos(Pitch)];
    R_z = [cos(Yaw)     sin(Yaw)      0;
          -sin(Yaw)     cos(Yaw)      0;
              0            0          1];
    J = (R_z'*R_y')*R_x';
end

== matlab function sim_all/Controller_mk4_v3/C_pos/C_pos_Y ==
  data: err_int output; pos input; vel output; k input; ctrl_vel_uncontrolled parameter; ctrl_int_bound_pos parameter
%% Azione proporzionale
function [err_int, vel] = fcn(pos, k, ctrl_vel_uncontrolled, ctrl_int_bound_pos)
    v = 0;
    err_int = 0;
    vel_des = ctrl_vel_uncontrolled;    % velocità impostata se 'lontani'
    brake_dist = 1/k*vel_des;           % distanza di frenata
    if pos >= brake_dist                % se ho spazio per frenare mantengo la velocità
        v = vel_des;
    end
    if pos <= -brake_dist               % lontani in direzione negativa
        v = -vel_des;
    end
    if  abs(pos) < brake_dist           % se è vicino il proporzionale gestisce la frenata
        v = k*pos;
    end
    vel = v;
    if abs(pos) < ctrl_int_bound_pos    % per il regime può essere utile una azione integrale
        err_int = pos;                  % err_int va ad un integratore
    end

== matlab function sim_all/PF/Particle Filter/Q_error/MATLAB Function4 ==
  data: Q input; Q_k_1 input; Q_k output; flag_AHRS input; flag_DVL input
function Q_k = fcn(Q, Q_k_1, flag_AHRS, flag_DVL)

    Q_k = Q;
    
    K=1;
    if flag_DVL == 1
       Q_k = Q_k_1 + K*diag([0,0,0,(0.012)^2,(0.012)^2,(0.012)^2]);
    end
    
    if flag_AHRS == 1
       Q_k = Q_k_1 + K*diag([0.0087, 0.0087, 0.0017,0,0,0]);  
    end
        
end

== matlab function sim_all/PF/Particle Filter/RICAMPIONAMENTO/MATLAB Function ==
  data: s input size=3 1000; s_new output size=3 1000; w input size=1 1000; w_new output size=1 1000; pulse input; nav_N_part parameter; n_eff output; n_eff_pulse output; en input
function [s_new, w_new,n_eff,n_eff_pulse] = fcn(s, w, pulse,nav_N_part,en)
coder.extrinsic('systematic_resample');
    s_new=s;
    w_new=w;    
    
    n_eff = 1/sum(w_new.^2);            %calcolo particelle effettive
    n_eff_pulse=nav_N_part*2/3*en;      %soglia per il ricampionamento

    %il resampling avviene in base ad un impulso per il ricampionamento
    %periodico e al numero delle particelle effettive
    if pulse==1 || n_eff < n_eff_pulse
       [s_new, w_new] = systematic_resample(s,w,nav_N_part);
    end 
        
    if n_eff < n_eff_pulse
       n_eff_pulse=1;
    else
       n_eff_pulse=0;
    end
end

== matlab function sim_all/PF/Gyro_check/MATLAB Function4 ==
  data: flag_gyro output; gyro_new input; gyro_now output; gyro_old input
function [flag_gyro, gyro_now] = fcn(gyro_new, gyro_old)

    if isnan(gyro_new(1,1)) || isnan(gyro_new(2,1)) || isnan(gyro_new(3,1))
        gyro_now = gyro_old;
        flag_gyro = 1;
        disp('Misura gyro non valida')
    else
        gyro_now = gyro_new;
        flag_gyro = 0;
    end  
end

== matlab function sim_all/PF/MATLAB Function ==
  data: u input; y output
function y = Wrap2pi(u)
y = [0;0;0];
coder.extrinsic('wrapToPi');
y = wrapToPi(u);
end

== matlab function sim_all/PF/NED2ECEF ==
  data: pos_es_NED input; pos_es_ECEF output; nav_lat0 parameter; nav_lon0 parameter; nav_h0 parameter


function pos_es_ECEF = pos_NED2ECEF(pos_es_NED,nav_lat0, nav_lon0, nav_h0)
     
    coder.extrinsic('evalin', 'wgs84Ellipsoid', 'ned2geodetic');
    pos_es_ECEF = zeros(3,1);
    depth = pos_es_NED(3); 
    
    [pos_es_ECEF(1),pos_es_ECEF(2),pos_es_ECEF(3)]= ned2geodetic(pos_es_NED(1),pos_es_NED(2),0,nav_lat0,nav_lon0,nav_h0,wgs84Ellipsoid);
    pos_es_ECEF(3) = depth;
end
